simulink model "final_ball_simulink_model"  (R2022b)
settings: Solver=VariableStepAuto  StartTime=0.0  StopTime=10.0  RelTol=1e-3
settings Model: Creator=User  LastModifiedBy=Wikian

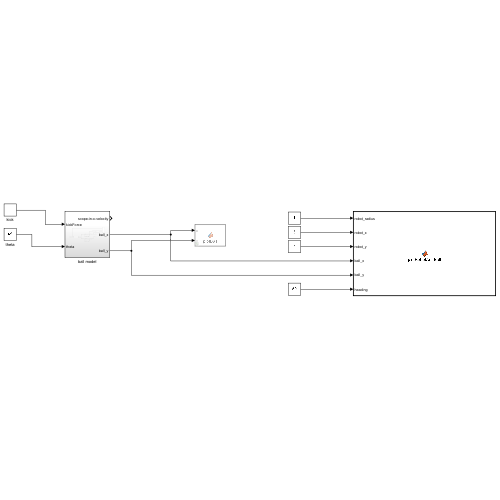
[thumbnail: Simulink's stored preview of the top-level diagram]
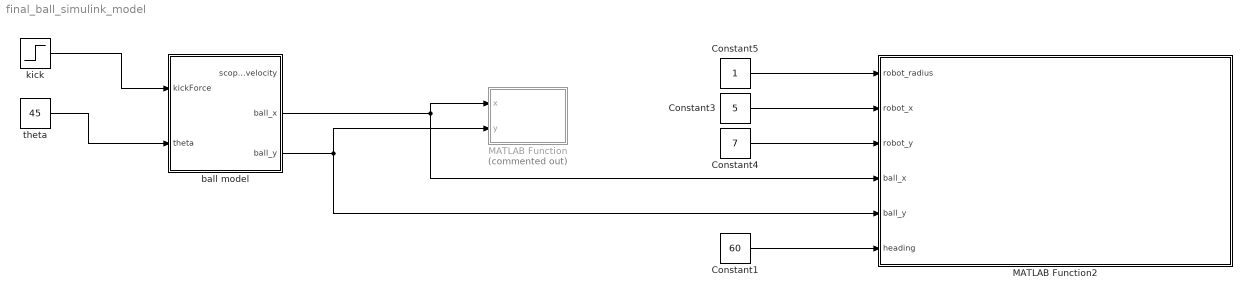
== system final_ball_simulink_model ==
  Constant1 : Constant  Value=60
  Constant3 : Constant  Value=5
  Constant4 : Constant  Value=7
  Constant5 : Constant
  MATLAB Function : MATLAB Function  Commented=on  TreatAsAtomicUnit=on
  MATLAB Function2 : MATLAB Function  InitFcn=|  TreatAsAtomicUnit=on
      | figure(1); 
      | clf;
      | hold on; 
      | grid on; 
      | axis([-45,45,-30,30]);
  ball model : Subsystem
  kick : Step  Time=0.1  Before=10  After=0  SampleTime=0
  theta : Constant  Value=45
  wires:
  kick/1 -> ball model/1(kickForce)
  ball model/2(ball_x) -> MATLAB Function/1(x), MATLAB Function2/4(ball_x)
  theta/1 -> ball model/2(theta)
  ball model/3(ball_y) -> MATLAB Function/2(y), MATLAB Function2/5(ball_y)
  Constant3/1 -> MATLAB Function2/2(robot_x)
  Constant4/1 -> MATLAB Function2/3(robot_y)
  Constant5/1 -> MATLAB Function2/1(robot_radius)
  Constant1/1 -> MATLAB Function2/6(heading)

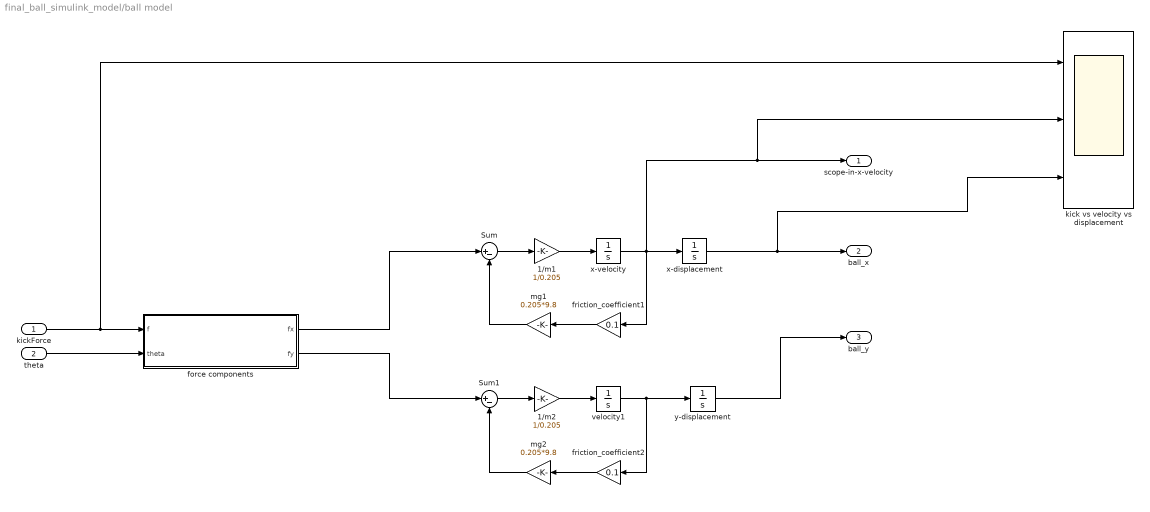
== system final_ball_simulink_model/ball model ==
  kickForce : Inport
  theta : Inport  Port=2
  1/m1 : Gain  Gain=1/0.205
  1/m2 : Gain  Gain=1/0.205
  Sum : Sum  Inputs=|+-
  Sum1 : Sum  Inputs=|+-
  force components : MATLAB Function  TreatAsAtomicUnit=on
  friction_coefficient1 : Gain  Gain=0.1
  friction_coefficient2 : Gain  Gain=0.1
  kick vs velocity vs displacement : Scope  NumInputPorts=3
  mg1 : Gain  Gain=0.205*9.8
  mg2 : Gain  Gain=0.205*9.8
  velocity1 : Integrator
  x-displacement : Integrator
  x-velocity : Integrator
  y-displacement : Integrator
  scope-in-x-velocity : Outport
  ball_x : Outport  Port=2
  ball_y : Outport  Port=3
  wires:
  velocity1/1 -> friction_coefficient2/1, y-displacement/1
  x-velocity/1 -> kick vs velocity vs displacement/2, scope-in-x-velocity/1, friction_coefficient1/1, x-displacement/1
  friction_coefficient2/1 -> mg2/1
  mg1/1 -> Sum/2
  Sum/1 -> 1/m1/1
  1/m2/1 -> velocity1/1
  friction_coefficient1/1 -> mg1/1
  force components/2(fy) -> Sum1/1
  Sum1/1 -> 1/m2/1
  1/m1/1 -> x-velocity/1
  force components/1(fx) -> Sum/1
  mg2/1 -> Sum1/2
  x-displacement/1 -> kick vs velocity vs displacement/3, ball_x/1
  theta/1 -> force components/2(theta)
  y-displacement/1 -> ball_y/1
  kickForce/1 -> kick vs velocity vs displacement/1, force components/1(f)

== matlab function final_ball_simulink_model/MATLAB Function ==
  data: x input; y input
function plotBall(x,y)
    figure(1); clf; hold on; grid on; axis([-30,30,-30,30]);
    plot(x,y,'Color','b','Marker','o');

== matlab function final_ball_simulink_model/ball model/force components ==
  data: f input; fx output; theta input; fy output
function [fx,fy] = getForceComponents(f, theta)
    
    fx = f*cos((theta*pi)/180);
    fy = f*sin((theta*pi)/180);

end

== matlab function final_ball_simulink_model/MATLAB Function2 ==
  data: robot_radius input; robot_x input; robot_y input; ball_x input; ball_y input; heading input
function plotRobotAndBall(robot_radius, robot_x, robot_y, ball_x, ball_y, heading)
    figure(1); 
    clf;
    hold on; 
    grid on; 
    axis([-45,45,-30,30]);

    theta = linspace(0, 2*pi, 360);   
    heading_line_length = 4; % L

    % equation of circle for representing robot
    robot_rep_x = robot_radius * cos(theta);
    robot_rep_y = robot_radius * sin(theta);

    heading_line_x = cos((heading*pi)/180) * heading_line_length;
    heading_line_y = sin((heading*pi)/180) * heading_line_length;

    % Draw circle around current location of robot
    plot((robot_rep_x + robot_x), (robot_rep_y + robot_y), 'Color', 'b');
   
    % Draw line from center of robot in the direction of the current heading
    line([robot_x,  robot_x + heading_line_x], [robot_y, robot_y + heading_line_y], 'color', 'b');
    
    % Plot ball
    plot(ball_x, ball_y,'Color','r','Marker','o')

    drawnow();

end
